simulink model "SWC_HALIN_CDD_type"  (R2021b)
(part 5 of 8)

  Demux1/221 -> Data Type Conversion253/1
  Demux1/88 -> Mux/8
  Demux1/201 -> Data Type Conversion233/1
  Demux1/208 -> Data Type Conversion248/1
  Demux1/107 -> Data Type Conversion139/1
  Data Type Conversion55/1 -> [VHAL_RRSensorFail_flg]  "VHAL_RRSensorFail_flg"
  Demux3/50 -> Data Type Conversion372/1
  Data Type Conversion723/1 -> Bitwise OR114/1
  Shift Arithmetic173/1 -> Bitwise OR77/2
  Data Type Conversion699/1 -> Shift Arithmetic269/1
  Shift Arithmetic111/1 -> Bitwise OR47/4
  Demux4/65 -> Data Type Conversion718/1
  Data Type Conversion250/1 -> [VHAL_FlashFGSChSta_enum]  "VHAL_FlashFGSChSta_enum"
  Data Type Conversion241/1 -> [VHAL_FlashREVentYSta_enum]  "VHAL_FlashREVentYSta_enum"
  Demux3/158 -> Data Type Conversion514/1
  Demux4/69 -> Data Type Conversion723/1
  Data Type Conversion67/1 -> Shift Arithmetic16/1
  Data Type Conversion249/1 -> [VHAL_FlashFGSAirIntSta_enum]  "VHAL_FlashFGSAirIntSta_enum"
  Demux3/24 -> Data Type Conversion339/1
  Demux4/200 -> Terminator55/1
  Data Type Conversion233/1 -> [VHAL_FlashTurnSwTSet457_enum]  "VHAL_FlashTurnSwTSet457_enum"
  Data Type Conversion232/1 -> [VHAL_FlashTurnSwTSet123_enum]  "VHAL_FlashTurnSwTSet123_enum"
  Shift Arithmetic287/1 -> Bitwise OR115/2
  Demux1/216 -> Data Type Conversion236/1
  Data Type Conversion139/1 -> [VHAL_FlashLockSetting_enum]  "VHAL_FlashLockSetting_enum"
  Shift Arithmetic275/1 -> Bitwise OR111/2
  Demux1/11 -> Data Type Conversion76/1
  Ground30/1 -> Data Type Conversion852/1
  Demux1/214 -> Data Type Conversion241/1
  Shift Arithmetic9/1 -> Bitwise OR3/2
  Data Type Conversion227/1 -> [VHAL_FlashAmbBrightnessSta2_enum]  "VHAL_FlashAmbBrightnessSta2_enum"
  Demux4/19 -> Data Type Conversion660/1
  Data Type Conversion617/1 -> Mux8/2
  Data Type Conversion245/1 -> [VHAL_FlashLEVentZSta_enum]  "VHAL_FlashLEVentZSta_enum"
  Demux4/196 -> Terminator43/1
  Demux4/75 -> Data Type Conversion730/1
  Data Type Conversion582/1 -> Mux7/3
  Demux4/250 -> Terminator_117/1
  Bitwise OR19/1 -> Data Type Conversion271/1
  Demux4/223 -> Terminator_90/1
  Demux4/36 -> Data Type Conversion681/1
  Data Type Conversion217/1 -> [VHAL_FlashAmbDimEN_enum]  "VHAL_FlashAmbDimEN_enum"
  Data Type Conversion733/1 -> Bitwise OR116/1
  Data Type Conversion832/1 -> [VHAL_FlashAirIntenZone1MSet4_enum]  "VHAL_FlashAirIntenZone1MSet4_enum"
  Data Type Conversion138/1 -> [VHAL_FlashFuelDoorPos_flg]  "VHAL_FlashFuelDoorPos_flg"
  Data Type Conversion792/1 -> Shift Arithmetic323/1
  Data Type Conversion609/1 -> Shift Arithmetic215/1
  Demux1/184 -> Data Type Conversion217/1
  Shift Arithmetic6/1 -> Bitwise OR2/2
  Demux1/204 -> Data Type Conversion244/1
  Demux1/198 -> Data Type Conversion230/1
  Demux4/214 -> Terminator_81/1
  Demux1/68 -> Data Type Conversion148/1
  Shift Arithmetic52/1 -> Bitwise OR24/2
  Data Type Conversion434/1 -> Bitwise OR51/1
  Demux1/66 -> Data Type Conversion146/1
  Demux1/218 -> Data Type Conversion250/1
  Bitwise OR114/1 -> Data Type Conversion727/1
  Demux1/56 -> Data Type Conversion893/1
  Demux4/171 -> Terminator32/1
  Demux1/19 -> Data Type Conversion65/1
  Data Type Conversion718/1 -> Bitwise OR113/1
  Demux1/149 -> Mux2/2
  Data Type Conversion178/1 -> Multiply2/1
  Demux4/27 -> Data Type Conversion670/1
  Data Type Conversion634/1 -> Shift Arithmetic230/1
  Data Type Conversion83/1 -> Shift Arithmetic15/1
  Demux1/77 -> Data Type Conversion157/1
  Data Type Conversion214/1 -> [VHAL_FlashAmbColorSta1_enum]  "VHAL_FlashAmbColorSta1_enum"
  Demux3/252 -> Data Type Conversion631/1
  Data Type Conversion671/1 -> Shift Arithmetic253/1
  Shift Arithmetic70/1 -> Bitwise OR31/3
  Demux4/30 -> Data Type Conversion674/1
  Data Type Conversion223/1 -> [VHAL_FlashAmbColorSta4_enum]  "VHAL_FlashAmbColorSta4_enum"
  Data Type Conversion218/1 -> [VHAL_FlashAmbLinkDriSta_enum]  "VHAL_FlashAmbLinkDriSta_enum"
  Shift Arithmetic30/1 -> Bitwise OR5/3
  Demux1/191 -> Data Type Conversion223/1
  Demux4/140 -> Data Type Conversion819/1
  Data Type Conversion221/1 -> [VHAL_FlashAmbColorSta2_enum]  "VHAL_FlashAmbColorSta2_enum"
  Data Type Conversion65/1 -> Bitwise OR8/1
  Demux1/7 -> Data Type Conversion72/1
  Demux1/193 -> Data Type Conversion225/1
  Data Type Conversion222/1 -> [VHAL_FlashAmbColorSta3_enum]  "VHAL_FlashAmbColorSta3_enum"
  Demux3/174 -> Data Type Conversion534/1
  Demux1/60 -> Data Type Conversion103/1
  Demux3/127 -> Data Type Conversion469/1
  Data Type Conversion256/1 -> Shift Arithmetic43/1
  Demux3/253 -> Data Type Conversion633/1
  Demux1/199 -> Data Type Conversion231/1
  Ground2/1 -> Data Type Conversion830/1
  Demux1/133 -> Mux1/2
  Data Type Conversion216/1 -> [VHAL_FlashAmbWelEN_enum]  "VHAL_FlashAmbWelEN_enum"
  Data Type Conversion598/1 -> Bitwise OR89/1
  Demux1/186 -> Data Type Conversion219/1
  Shift Arithmetic83/1 -> Bitwise OR36/3
  Data Type Conversion551/1 -> Shift Arithmetic181/1
  Demux1/2 -> Data Type Conversion64/1
  Data Type Conversion60/1 -> [VHAL_LFWheelPSW_raw8]  "VHAL_LFWheelPSW_raw8"
  Data Type Conversion215/1 -> [VHAL_FlashAmbFunEN_enum]  "VHAL_FlashAmbFunEN_enum"
  Demux3/153 -> Data Type Conversion508/1
  Demux1/130 -> Data Type Conversion192/1
  Data Type Conversion225/1 -> [VHAL_FlashAmbColorSta7_enum]  "VHAL_FlashAmbColorSta7_enum"
  Shift Arithmetic69/1 -> Bitwise OR31/2
  Data Type Conversion768/1 -> convert_out24/1
  Data Type Conversion104/1 -> [VHAL_Flashchkdatavalid_enum]  "VHAL_Flashchkdatavalid_enum"
  Demux3/147 -> Data Type Conversion499/1
  Data Type Conversion230/1 -> [VHAL_FlashAmbBrightnessSta5_enum]  "VHAL_FlashAmbBrightnessSta5_enum"
  Data Type Conversion120/1 -> [VHAL_DIDFlashDKCKey_raw8]
  Demux1/187 -> Data Type Conversion220/1
  Data Type Conversion129/1 -> [VHAL_FlashACForceOFF_flg]  "VHAL_FlashACForceOFF_flg"
  Demux1/185 -> Data Type Conversion218/1
  Data Type Conversion716/1 -> Shift Arithmetic280/1
  Ground33/1 -> Data Type Conversion862/1
  Shift Arithmetic255/1 -> Bitwise OR104/3
  Ground28/1 -> Data Type Conversion850/1
  Demux1/195 -> Data Type Conversion227/1
  Bitwise OR102/1 -> Data Type Conversion667/1
  Data Type Conversion797/1 -> Shift Arithmetic326/1
  Shift Arithmetic321/1 -> Bitwise OR126/3
  Data Type Conversion220/1 -> [VHAL_FlashAmbODAEN_enum]  "VHAL_FlashAmbODAEN_enum"
  Demux3/15 -> Data Type Conversion328/1
  Data Type Conversion531/1 -> Shift Arithmetic169/1
  Data Type Conversion62/1 -> [VHAL_RFPindi_enum]  "VHAL_RFPindi_enum"
  Data Type Conversion859/1 -> [VHAL_FlashCREVentZStaSet2_enum]  "VHAL_FlashCREVentZStaSet2_enum"
  Bitwise OR31/1 -> Data Type Conversion340/1
  Demux1/207 -> Data Type Conversion247/1
  Demux1/189 -> Data Type Conversion221/1
  Bitwise OR10/1 -> Data Type Conversion891/1
  Demux4/8 -> Data Type Conversion646/1
  Demux1/173 -> Mux3/10
  Data Type Conversion307/1 -> [VHAL_FlashCLRTIME_min]  "VHAL_FlashCLRTIME_min"
  Demux1/176 -> Mux3/13
  Demux4/23 -> Data Type Conversion665/1
  Data Type Conversion61/1 -> [VHAL_RRWheelPSW_raw8]  "VHAL_RRWheelPSW_raw8"
  Data Type Conversion209/1 -> [VHAL_DIDFlashTireSize_raw8]  "VHAL_DIDFlashTireSize_raw8"
  Demux1/180 -> Data Type Conversion211/1
  Bitwise OR112/1 -> Data Type Conversion717/1
  Demux1/175 -> Mux3/12
  Demux4/91 -> Data Type Conversion750/1
  Data Type Conversion210/1 -> [VHAL_DIDFlashAPSFunConfig_raw8]  "VHAL_DIDFlashAPSFunConfig_raw8"
  Demux3/92 -> Data Type Conversion425/1
  Demux1/212 -> Data Type Conversion239/1
  Demux3/74 -> Data Type Conversion402/1
  Demux3/81 -> Data Type Conversion411/1
  Shift Arithmetic78/1 -> Bitwise OR34/2
  Ground23/1 -> Data Type Conversion860/1
  Mux10/1 -> Data Type Conversion807/1
  Bitwise OR82/1 -> Data Type Conversion567/1
  Shift Arithmetic107/1 -> Bitwise OR44/3
  Mux4/1 -> Data Type Conversion813/1
  Demux3/44 -> Data Type Conversion365/1
  Demux3/45 -> Data Type Conversion366/1
  Shift Arithmetic186/1 -> Bitwise OR81/3
  Bitwise OR118/1 -> Data Type Conversion747/1
  convert_out22/1 -> [VHAL_FlashAvgBattTempOFFR_C]  "VHAL_FlashAvgBattTempOFFR_C"
  Demux3/62 -> Data Type Conversion387/1
  Demux3/57 -> Data Type Conversion381/1
  Demux4/242 -> Terminator_109/1
  Data Type Conversion760/1 -> Shift Arithmetic306/1
  Shift Arithmetic322/1 -> Bitwise OR126/4
  Shift Arithmetic85/1 -> Bitwise OR37/2
  Shift Arithmetic190/1 -> Bitwise OR82/4
  Shift Arithmetic91/1 -> Bitwise OR39/2
  Data Type Conversion436/1 -> Shift Arithmetic128/1
  Data Type Conversion40/1 -> Shift Arithmetic82/1
  Data Type Conversion150/1 -> Shift Arithmetic7/1
  Data Type Conversion378/1 -> convert_out8/1
  Data Type Conversion610/1 -> Shift Arithmetic216/1
  Shift Arithmetic283/1 -> Bitwise OR113/4
  Shift Arithmetic108/1 -> Bitwise OR44/4
  Shift Arithmetic118/1 -> Bitwise OR45/2
  Demux4/130 -> Data Type Conversion798/1
  Demux1/120 -> Data Type Conversion180/1
  Demux4/54 -> Data Type Conversion704/1
  Demux1/197 -> Data Type Conversion229/1
  Shift Arithmetic193/1 -> Bitwise OR83/4
  Shift Arithmetic96/1 -> Bitwise OR40/4
  Data Type Conversion461/1 -> Shift Arithmetic139/1
  Demux3/23 -> Data Type Conversion338/1
  Data Type Conversion757/1 -> Mux11/6
  Data Type Conversion399/1 -> Bitwise OR44/1
  Shift Arithmetic313/1 -> Bitwise OR123/4
  Demux1/54 -> Data Type Conversion51/1
  Shift Arithmetic241/1 -> Bitwise OR99/4
  Demux4/5 -> Data Type Conversion643/1
  Demux1/1 -> Data Type Conversion63/1
  Data Type Conversion377/1 -> Shift Arithmetic93/1
  Demux3/102 -> Data Type Conversion437/1
  Data Type Conversion691/1 -> Shift Arithmetic265/1
  Shift Arithmetic82/1 -> Bitwise OR36/2
  Shift Arithmetic131/1 -> Bitwise OR52/3
  Data Type Conversion252/1 -> [VHAL_FlashWalkOutLkEN_enum]  "VHAL_FlashWalkOutLkEN_enum"
  Demux1/206 -> Data Type Conversion246/1
  Data Type Conversion841/1 -> [VHAL_FlashFGSAirIntStaSet457_enum]  "VHAL_FlashFGSAirIntStaSet457_enum"
  Data Type Conversion387/1 -> Shift Arithmetic99/1
  Shift Arithmetic86/1 -> Bitwise OR37/3
  Shift Arithmetic145/1 -> Bitwise OR61/2
  Data Type Conversion714/1 -> Shift Arithmetic278/1
  Demux1/136 -> Mux1/5
  Data Type Conversion296/1 -> Shift Arithmetic49/1
  Shift Arithmetic87/1 -> Bitwise OR37/4
  Data Type Conversion254/1 -> Bitwise OR15/1
  Demux1/36 -> Data Type Conversion53/1
  Data Type Conversion855/1 -> [VHAL_FlashREVentZStaSet3_enum]  "VHAL_FlashREVentZStaSet3_enum"
  Data Type Conversion46/1 -> [VHAL_LRP20_raw8]  "VHAL_LRP20_raw8"
  Demux1/226 -> Data Type Conversion258/1
  Data Type Conversion719/1 -> Shift Arithmetic281/1
  Bitwise OR14/1 -> Data Type Conversion178/1
  Data Type Conversion854/1 -> [VHAL_FlashREVentZStaSet2_enum]  "VHAL_FlashREVentZStaSet2_enum"
  Data Type Conversion394/1 -> Bitwise OR43/1
  Shift Arithmetic296/1 -> Bitwise OR118/2
  Bitwise OR37/1 -> Data Type Conversion43/1
  Data Type Conversion690/1 -> Shift Arithmetic264/1
  Demux3/170 -> Data Type Conversion529/1
  Data Type Conversion791/1 -> Bitwise OR127/1
  Data Type Conversion248/1 -> [VHAL_FlashCREVentZSta_enum]  "VHAL_FlashCREVentZSta_enum"
  Demux4/219 -> Terminator_86/1
  Shift Arithmetic99/1 -> Bitwise OR41/4
  Data Type Conversion683/1 -> Bitwise OR106/1
  Demux4/127 -> Data Type Conversion794/1
  Shift Arithmetic150/1 -> Bitwise OR66/2
  Bitwise OR38/1 -> Data Type Conversion368/1
  Data Type Conversion244/1 -> [VHAL_FlashLEVentModeSta_enum]  "VHAL_FlashLEVentModeSta_enum"
  Shift Arithmetic90/1 -> Bitwise OR38/4
  Shift Arithmetic103/1 -> Bitwise OR43/2
  Shift Arithmetic105/1 -> Bitwise OR43/4
  Shift Arithmetic270/1 -> Bitwise OR109/3
  Demux3/150 -> Data Type Conversion503/1
  Data Type Conversion395/1 -> Shift Arithmetic103/1
  Data Type Conversion511/1 -> Shift Arithmetic157/1
  Demux1/16 -> Data Type Conversion81/1
  Shift Arithmetic326/1 -> Bitwise OR128/2
  Shift Arithmetic214/1 -> Bitwise OR90/4
  Demux3/231 -> Data Type Conversion605/1
  Multiply2/1 -> Data Type Conversion168/1
  Data Type Conversion890/1 -> [VHAL_FlashJugKeepUnLZone_flg]  "VHAL_FlashJugKeepUnLZone_flg"
  Data Type Conversion84/1 -> [VHAL_FlashChkLFID_raw]  "VHAL_FlashChkLFID_raw"
  Data Type Conversion253/1 -> [VHAL_FlashWalkInUnLkEN_enum]  "VHAL_FlashWalkInUnLkEN_enum"
  Bitwise OR1/1 -> Data Type Conversion160/1
  Shift Arithmetic94/1 -> Bitwise OR40/2
  Data Type Conversion353/1 -> Shift Arithmetic79/1
  Demux1/205 -> Data Type Conversion245/1
  Demux3/34 -> Data Type Conversion352/1
  Demux1/91 -> Data Type Conversion123/1
  Data Type Conversion157/1 -> Shift Arithmetic36/1
  Data Type Conversion373/1 -> convert_out7/1
  Shift Arithmetic14/1 -> Bitwise OR7/3
  Demux1/220 -> Data Type Conversion252/1
  Demux1/50 -> Data Type Conversion48/1
  Demux3/37 -> Data Type Conversion356/1
  Demux1/202 -> Data Type Conversion234/1
  Selector3/1 -> Demux4/1
  Data Type Conversion506/1 -> Shift Arithmetic154/1
  Demux4/98 -> Data Type Conversion759/1
  Data Type Conversion356/1 -> Bitwise OR35/1
  Shift Arithmetic242/1 -> Bitwise OR100/2
  Demux3/38 -> Data Type Conversion357/1
  Demux3/66 -> Data Type Conversion392/1
  Shift Arithmetic3/1 -> Bitwise OR12/3
  Data Type Conversion885/1 -> [VHAL_FlashSettempZon1Set2_enum]  "VHAL_FlashSettempZon1Set2_enum"
  Shift Arithmetic81/1 -> Bitwise OR35/2
  Shift Arithmetic218/1 -> Bitwise OR92/2
  Demux1/51 -> Data Type Conversion50/1
  Data Type Conversion432/1 -> Shift Arithmetic126/1
  Demux4/107 -> Data Type Conversion770/1
  Demux1/73 -> Data Type Conversion153/1
  Shift Arithmetic80/1 -> Bitwise OR34/4
  Demux3/18 -> Data Type Conversion332/1
  Data Type Conversion153/1 -> Shift Arithmetic9/1
  Shift Arithmetic110/1 -> Bitwise OR47/3
  Data Type Conversion881/1 -> [VHAL_FlashCREVentYStaSet4_enum]  "VHAL_FlashCREVentYStaSet4_enum"
  Shift Arithmetic71/1 -> Bitwise OR31/4
  Data Type Conversion703/1 -> Bitwise OR110/1
  Data Type Conversion182/1 -> [VHAL_FlashCTDLockSW_flg]  "VHAL_FlashCTDLockSW_flg"
  Bitwise OR27/1 -> Data Type Conversion320/1
  Demux4/68 -> Data Type Conversion721/1
  Data Type Conversion346/1 -> Bitwise OR33/1
  Shift Arithmetic77/1 -> Bitwise OR33/4
  Demux4/40 -> Data Type Conversion686/1
  Bitwise OR15/1 -> Data Type Conversion259/1
  Demux4/57 -> Data Type Conversion708/1
  Demux4/218 -> Terminator_85/1
  Bitwise OR121/1 -> Data Type Conversion762/1
  Demux1/178 -> Mux3/15
  Bitwise OR52/1 -> Data Type Conversion439/1
  Data Type Conversion332/1 -> Shift Arithmetic66/1
  Demux3/32 -> Data Type Conversion349/1
  Demux3/27 -> Data Type Conversion343/1
  Data Type Conversion468/1 -> Mux4/3
  Data Type Conversion325/1 -> [VHAL_FlashPSAL_sec]  "VHAL_FlashPSAL_sec"
  convert_out10/1 -> [VHAL_FlashTGEOVCR_kWh]  "VHAL_FlashTGEOVCR_kWh"
  Data Type Conversion871/1 -> [VHAL_FlashCLEVentYStaSet4_enum]  "VHAL_FlashCLEVentYStaSet4_enum"
  Data Type Conversion366/1 -> Shift Arithmetic86/1
  Data Type Conversion336/1 -> Bitwise OR31/1
  Shift Arithmetic56/1 -> Bitwise OR26/4
  Data Type Conversion601/1 -> Shift Arithmetic211/1
  Shift Arithmetic304/1 -> Bitwise OR120/4
  Data Type Conversion344/1 -> Shift Arithmetic74/1
  Demux4/1 -> Data Type Conversion638/1
  Shift Arithmetic141/1 -> Bitwise OR57/2
  Data Type Conversion243/1 -> [VHAL_FlashREVentModeSta_enum]  "VHAL_FlashREVentModeSta_enum"
  Data Type Conversion681/1 -> Shift Arithmetic259/1
  Shift Arithmetic135/1 -> Bitwise OR53/4
  Data Type Conversion357/1 -> Shift Arithmetic81/1
  Data Type Conversion312/1 -> Shift Arithmetic54/1
  Shift Arithmetic187/1 -> Bitwise OR81/4
  Shift Arithmetic62/1 -> Bitwise OR28/4
  Bitwise OR62/1 -> Data Type Conversion483/1
  Demux3/9 -> Data Type Conversion321/1
  Demux3/1 -> Data Type Conversion311/1
  Shift Arithmetic59/1 -> Bitwise OR27/4
  Data Type Conversion331/1 -> Bitwise OR30/1
  Data Type Conversion316/1 -> Bitwise OR27/1
  Shift Arithmetic189/1 -> Bitwise OR82/3
  Shift Arithmetic247/1 -> Bitwise OR101/4
  Data Type Conversion684/1 -> Shift Arithmetic260/1
  Demux3/211 -> Data Type Conversion580/1
  Data Type Conversion484/1 -> Bitwise OR63/1
  Data Type Conversion319/1 -> Shift Arithmetic59/1
  Demux3/10 -> Data Type Conversion322/1
  Demux3/59 -> Data Type Conversion384/1
  Demux4/230 -> Terminator_97/1
  Data Type Conversion101/1 -> [VHAL_RRWheelTemp_C]  "VHAL_RRWheelTemp_C"
  Demux4/102 -> Data Type Conversion764/1
  Shift Arithmetic122/1 -> Bitwise OR46/3
  Shift Arithmetic72/1 -> Bitwise OR32/2
  Shift Arithmetic106/1 -> Bitwise OR44/2
  Shift Arithmetic256/1 -> Bitwise OR104/4
  Data Type Conversion314/1 -> Shift Arithmetic56/1
  Demux1/99 -> FlashAirIntenZone1M_Verify/1(In1)
  Demux3/145 -> Data Type Conversion496/1
  Data Type Conversion226/1 -> [VHAL_FlashAmbBrightnessSta1_enum]  "VHAL_FlashAmbBrightnessSta1_enum"
  Data Type Conversion445/1 -> convert_out19/1
  Demux3/54 -> Data Type Conversion377/1
  Demux1/252 -> Data Type Conversion303/1
  Shift Arithmetic31/1 -> Bitwise OR5/4
  Data Type Conversion653/1 -> Bitwise OR100/1
  Data Type Conversion306/1 -> Shift Arithmetic52/1
  Data Type Conversion308/1 -> Bitwise OR25/1
  Bitwise OR13/1 -> Data Type Conversion173/1
  Data Type Conversion349/1 -> Shift Arithmetic77/1
  Data Type Conversion161/1 -> [VHAL_FlashS2ID_raw]  "VHAL_FlashS2ID_raw"
  Demux3/19 -> Data Type Conversion333/1
  Demux3/245 -> Data Type Conversion623/1
  Demux3/68 -> Data Type Conversion395/1
  Shift Arithmetic205/1 -> Bitwise OR87/4
  Bitwise OR105/1 -> Data Type Conversion682/1
  Demux3/120 -> Data Type Conversion458/1
  Data Type Conversion301/1 -> [VHAL_FlashCLRDIST_km]  "VHAL_FlashCLRDIST_km"
  Data Type Conversion674/1 -> Shift Arithmetic254/1
  Shift Arithmetic53/1 -> Bitwise OR25/2
  Shift Arithmetic42/1 -> Bitwise OR14/4
  [HAL_NvmReadData_raw] -> Selector2/1
  Demux1/230 -> Data Type Conversion264/1
  Shift Arithmetic2/1 -> Bitwise OR1/3
  Shift Arithmetic29/1 -> Bitwise OR5/2
  Shift Arithmetic55/1 -> Bitwise OR26/3
  Data Type Conversion121/1 -> [VHAL_FlashACModeSet123_enum]  "VHAL_FlashACModeSet123_enum"
  Data Type Conversion74/1 -> Shift Arithmetic30/1
  Data Type Conversion655/1 -> Shift Arithmetic243/1
  Ground57/1 -> Data Type Conversion885/1
  Data Type Conversion92/1 -> Shift Arithmetic23/1
  Demux3/106 -> Data Type Conversion443/1
  Data Type Conversion123/1 -> [VHAL_FlashFoot_enum]  "VHAL_FlashFoot_enum"
  Demux1/30 -> Data Type Conversion96/1
  Demux4/10 -> Data Type Conversion649/1
  Bitwise OR28/1 -> Data Type Conversion325/1
  Data Type Conversion348/1 -> Shift Arithmetic76/1
  Shift Arithmetic36/1 -> Bitwise OR12/2
  Bitwise OR86/1 -> Data Type Conversion587/1
  Demux1/253 -> Data Type Conversion305/1
  Data Type Conversion347/1 -> Shift Arithmetic75/1
  Demux3/192 -> Data Type Conversion556/1
  Bitwise OR113/1 -> Data Type Conversion722/1
  Demux3/132 -> Data Type Conversion476/1
  Data Type Conversion845/1 -> [VHAL_FlashLEVentZStaSet3_enum]  "VHAL_FlashLEVentZStaSet3_enum"
  Demux1/254 -> Data Type Conversion306/1
  Data Type Conversion309/1 -> Shift Arithmetic53/1
  Data Type Conversion586/1 -> Shift Arithmetic202/1
  [HAL_NvmReadData_raw] -> Selector1/1
  Demux1/147 -> Mux1/16
  Data Type Conversion638/1 -> Bitwise OR97/1
  Demux4/180 -> Terminator27/1
  Data Type Conversion146/1 -> Shift Arithmetic2/1
  Data Type Conversion631/1 -> Shift Arithmetic229/1
  Data Type Conversion322/1 -> Shift Arithmetic60/1
  convert_out24/1 -> [VHAL_FlashMAXBATTEMPL_C]  "VHAL_FlashMAXBATTEMPL_C"
  Bitwise OR68/1 -> Data Type Conversion501/1
  Data Type Conversion587/1 -> Mux7/4
  Demux1/228 -> Data Type Conversion262/1
  Data Type Conversion133/1 -> [VHAL_FlashsigSetTempZon1St_C]  "VHAL_FlashsigSetTempZon1St_C"
  Data Type Conversion176/1 -> Shift Arithmetic41/1
  Demux1/3 -> Data Type Conversion66/1
  Demux3/6 -> Data Type Conversion317/1
  Bitwise OR25/1 -> Data Type Conversion310/1
  Ground56/1 -> Data Type Conversion884/1
  Shift Arithmetic11/1 -> Bitwise OR3/4
  Shift Arithmetic74/1 -> Bitwise OR32/4
  Demux4/217 -> Terminator_84/1
  Demux4/185 -> Terminator62/1
  Data Type Conversion647/1 -> [VHAL_FlashRESSTIMESOCCHGRNGR7_s]
  Bitwise OR79/1 -> Data Type Conversion552/1
  Data Type Conversion304/1 -> [VHAL_FlashMILTIME_min]  "VHAL_FlashMILTIME_min"
  Shift Arithmetic75/1 -> Bitwise OR33/2
  Shift Arithmetic154/1 -> Bitwise OR70/2
  Data Type Conversion352/1 -> Shift Arithmetic78/1
  Demux4/225 -> Terminator_92/1
  Demux3/129 -> Data Type Conversion472/1
  Bitwise OR22/1 -> Data Type Conversion301/1
  Shift Arithmetic93/1 -> Bitwise OR39/4
  Demux4/67 -> Data Type Conversion720/1
  Demux1/232 -> Data Type Conversion268/1
  Data Type Conversion426/1 -> Shift Arithmetic116/1
  Demux1/122 -> Data Type Conversion182/1
  Demux3/36 -> Data Type Conversion354/1
  Demux3/223 -> Data Type Conversion595/1
  Data Type Conversion236/1 -> [VHAL_FlashCREVentYSta_enum]  "VHAL_FlashCREVentYSta_enum"
  Data Type Conversion302/1 -> Bitwise OR23/1
  Data Type Conversion36/1 -> [VHAL_FlashWARMUPS_cnt]  "VHAL_FlashWARMUPS_cnt"
  Bitwise OR30/1 -> Data Type Conversion335/1
  Data Type Conversion847/1 -> [VHAL_FlashLEVentZStaSet5_enum]  "VHAL_FlashLEVentZStaSet5_enum"
  Data Type Conversion738/1 -> Bitwise OR117/1
  Demux1/248 -> Data Type Conversion36/1
  Shift Arithmetic17/1 -> Bitwise OR8/3
  Demux4/191 -> Terminator38/1
  Shift Arithmetic28/1 -> Bitwise OR11/2
  Demux4/13 -> Data Type Conversion653/1
  Mux1/1 -> Data Type Conversion208/1
  Bitwise OR23/1 -> Data Type Conversion304/1
  Demux1/114 -> Data Type Conversion171/1
  Data Type Conversion807/1 -> [VHAL_FlashRESSTIMESOCOFFRNGR_s]  "VHAL_FlashRESSTIMESOCOFFRNGR_s"
  Demux1/159 -> Mux2/12
  Data Type Conversion299/1 -> Bitwise OR22/1
  Demux1/210 -> Data Type Conversion237/1
  Data Type Conversion136/1 -> [VHAL_FlashMFSWTri_flg]  "VHAL_FlashMFSWTri_flg"
  Demux1/247 -> Data Type Conversion296/1
  Data Type Conversion662/1 -> Mux9/3
  Shift Arithmetic44/1 -> Bitwise OR16/2
  Shift Arithmetic48/1 -> Bitwise OR20/2
  Data Type Conversion408/1 -> convert_out14/1
  Data Type Conversion219/1 -> [VHAL_FlashAmbPwrWarnEN_enum]  "VHAL_FlashAmbPwrWarnEN_enum"
  Data Type Conversion37/1 -> [VHAL_DIDFlashTurnLampFRThreCurr_raw8]  "VHAL_DIDFlashTurnLampFRThreCurr_raw8"
  Shift Arithmetic204/1 -> Bitwise OR87/3
  Data Type Conversion472/1 -> Bitwise OR59/1
  Data Type Conversion523/1 -> Bitwise OR74/1
  Demux1/37 -> Data Type Conversion54/1
  Demux3/176 -> Data Type Conversion536/1
  Data Type Conversion709/1 -> Shift Arithmetic275/1
  Data Type Conversion147/1 -> Shift Arithmetic5/1
  Demux1/240 -> Data Type Conversion34/1
  Shift Arithmetic60/1 -> Bitwise OR28/2
  Data Type Conversion172/1 -> Shift Arithmetic39/1
  Data Type Conversion334/1 -> Shift Arithmetic68/1
  Shift Arithmetic22/1 -> Bitwise OR9/3
  Demux1/41 -> Data Type Conversion59/1
  Data Type Conversion422/1 -> Shift Arithmetic114/1
  Demux1/183 -> Data Type Conversion216/1
  Ground1/1 -> DIDGet_List/4(VHAL_DIDFlashDynoMode_raw8)
  [VHAL_DIDFlashDKCKey_raw8] -> DIDGet_List/3(VHAL_DIDFlashDKCKey_raw8)
  [VHAL_DIDFlashXWDMode_raw8] -> DIDGet_List/2(VHAL_DIDFlashXWDMode_raw8)
  [VHAL_DIDFlashWipRLSCmdHoldFilter_raw8] -> DIDGet_List/13(VHAL_DIDFlashWipRLSCmdHoldFilter_raw8)
  [VHAL_DIDFlashAutoWipHSpdEN_raw8] -> DIDGet_List/12(VHAL_DIDFlashAutoWipHSpdEN_raw8)
  [VHAL_DIDFlashDRLDis_raw8] -> DIDGet_List/11(VHAL_DIDFlashDRLDis_raw8)
  [VHAL_DIDFlashAutoLock_raw8] -> DIDGet_List/10(VHAL_DIDFlashAutoLock_raw8)
  [VHAL_DIDFlashFMHTimer_raw8] -> DIDGet_List/9(VHAL_DIDFlashFMHTimer_raw8)
  [BHAL_DIDGetData_raw] -> DIDGet_List/1(BHAL_DIDGetData_raw)
  [VHAL_DIDFlashTurnLampRLThreCurr_raw8] -> DIDGet_List/8(VHAL_DIDFlashTurnLampRLThreCurr_raw8)
  [VHAL_DIDFlashTurnLampFLThreCurr_raw8] -> DIDGet_List/7(VHAL_DIDFlashTurnLampFLThreCurr_raw8)
  [VHAL_DIDFlashTurnLampRRThreCurr_raw8] -> DIDGet_List/6(VHAL_DIDFlashTurnLampRRThreCurr_raw8)
  DIDGet_List/1(BHAL_DIDOrigOutput_raw8) -> [BHAL_DIDOrigOutput_raw8]
  [VHAL_DIDFlashTestGroup_raw8] -> DIDGet_List/19(VHAL_DIDFlashTestGroup_raw8)
  [VHAL_DIDFlashTireSize_raw8] -> DIDGet_List/16(VHAL_DIDFlashTireSize_raw8)
  [VHAL_DIDFlashTurnLampFRThreCurr_raw8] -> DIDGet_List/5(VHAL_DIDFlashTurnLampFRThreCurr_raw8)
  [VHAL_DIDFlashUSSConfig_raw8] -> DIDGet_List/15(VHAL_DIDFlashUSSConfig_raw8)
  [VHAL_DIDFlashAPSFunConfig_raw8] -> DIDGet_List/17(VHAL_DIDFlashAPSFunConfig_raw8)
  [VHAL_DIDFlashWipRLSCmdCutFilter_raw8] -> DIDGet_List/14(VHAL_DIDFlashWipRLSCmdCutFilter_raw8)
  [VHAL_DIDFlashOBDReq_raw8] -> DIDGet_List/18(VHAL_DIDFlashOBDReq_raw8)
